simulink model "DLCReferenceApplication"  (R2020b)
settings: Solver=ode23tb  StartTime=0.0  StopTime=25  FixedStep=.001  RelTol=5e-3  EnableMultiTasking=on
StartFcn:
  | %tic
StopFcn:
  | %toc
model workspace (MAT data in the model file):
  DLCXref = [0 7.23 7.5 18 33 33.5 45 50 60]
  DLCYref = [0 0 -4.5 -4 -3.75 1.5 1.25 0 0]
  Downshift_Speeds = [9.5625 12.9375 16.3125 19.6875 23.0625 26.4375 29.8125 33.1875 36.5625 39.9375 43.3125 46.6875 ... (28 elements, 4x7)]
  EngRevLim = 7000
  Pedal_Positions = [0.1 0.4 0.5 0.9]
  Upshift_Speeds = [12.9375 16.3125 19.6875 33 26.4375 29.8125 33.1875 52.5 39.9375 43.3125 46.6875 77.25 ... (28 elements, 4x7)]
  VEH : object (value not decoded)
values from neighbouring files (symbols this model uses):
  L = 3.705    [AOTDataDictionary.sldd]
symbols that are objects in the model workspace (value not decoded): VEH
libraries: simulink x11, autolibutils x4, sim3dlib x2, pid_lib x1, autolibshared x1, vehdynlibdriver x1, vehdynlibscenariocommon x1, vehdynlibsens x1, sim3dautolib x1, vehdynlibviscommon x1
(part 3 of 3)

== system DLCReferenceApplication/Controllers/Transmission Controller/Transmission Controller/TCM/TCM Shift Controller/calc ==
  note: Determine if next gear will be
      | higher or lower than current gear
  gear : Inport
  pedal : Inport  Port=2
  speed : Inport  Port=3
  f : TriggerPort  TriggerType=function-call  VariantControl=Variant  StatesWhenEnabling=reset
      settings: CopyFcn=Stateflow.SLINSF.SimulinkMan.removeBlockPreDeleteFcn  PreDeleteFcn=Stateflow.SLINSF.SimulinkMan.unsafePredeleteFcn
  Add1 : Sum  Inputs=+-
  Add3 : Sum  Inputs=+-
  Add4 : Sum  Inputs=+-
  Calculate Upshift Threshold : Lookup_n-D  BreakpointsForDimension1=Pedal_Positions  BreakpointsForDimension2=1:7  Table=Upshift_Speeds  ExtrapMethod=Clip  UseLastTableValue=on  InternalRulePriority=Speed  RndMeth=Simplest  InputSameDT=on
      settings: InputPortMap=u0,u1
  Calculate Downshift Threshold : Lookup_n-D  BreakpointsForDimension1=Pedal_Positions  BreakpointsForDimension2=2:8  Table=Downshift_Speeds  ExtrapMethod=Clip  UseLastTableValue=on  InternalRulePriority=Speed  RndMeth=Simplest  InputSameDT=on
      settings: InputPortMap=u0,u1
  SpdThr : Outport  VectorParamsAs1DForOutWhenUnconnected=off
  wires:
  pedal/1 -> Calculate Downshift Threshold/1, Calculate Upshift Threshold/1
  gear/1 -> Calculate Downshift Threshold/2, Calculate Upshift Threshold/2
  Calculate Downshift Threshold/1 -> Add3/2
  Calculate Upshift Threshold/1 -> Add1/1
  speed/1 -> Add1/2, Add3/1
  Add1/1 -> Add4/1
  Add3/1 -> Add4/2
  Add4/1 -> SpdThr/1

== system DLCReferenceApplication/Controllers/Transmission Controller/Transmission Controller/TCM/TCM Shift Controller/calc_down ==
  gear : Inport
  pedal : Inport  Port=2
  f : TriggerPort  TriggerType=function-call  VariantControl=Variant  StatesWhenEnabling=reset
      settings: CopyFcn=Stateflow.SLINSF.SimulinkMan.removeBlockPreDeleteFcn  PreDeleteFcn=Stateflow.SLINSF.SimulinkMan.unsafePredeleteFcn
  Calculate Downshift Threshold : Lookup_n-D  BreakpointsForDimension1=Pedal_Positions  BreakpointsForDimension2=2:8  Table=Downshift_Speeds  ExtrapMethod=Clip  UseLastTableValue=on  InternalRulePriority=Speed  RndMeth=Simplest  InputSameDT=on
      settings: InputPortMap=u0,u1
  down_th : Outport  VectorParamsAs1DForOutWhenUnconnected=off
  wires:
  Calculate Downshift Threshold/1 -> down_th/1
  gear/1 -> Calculate Downshift Threshold/2
  pedal/1 -> Calculate Downshift Threshold/1

== system DLCReferenceApplication/Controllers/Transmission Controller/Transmission Controller/TCM/TCM Shift Controller/calc_up ==
  gear : Inport
  pedal : Inport  Port=2
  f : TriggerPort  TriggerType=function-call  VariantControl=Variant  StatesWhenEnabling=reset
      settings: CopyFcn=Stateflow.SLINSF.SimulinkMan.removeBlockPreDeleteFcn  PreDeleteFcn=Stateflow.SLINSF.SimulinkMan.unsafePredeleteFcn
  Calculate Upshift Threshold : Lookup_n-D  BreakpointsForDimension1=Pedal_Positions  BreakpointsForDimension2=1:7  Table=Upshift_Speeds  ExtrapMethod=Clip  UseLastTableValue=on  InternalRulePriority=Speed  RndMeth=Simplest  InputSameDT=on
      settings: InputPortMap=u0,u1
  up_th : Outport  VectorParamsAs1DForOutWhenUnconnected=off
  wires:
  Calculate Upshift Threshold/1 -> up_th/1
  pedal/1 -> Calculate Upshift Threshold/1
  gear/1 -> Calculate Upshift Threshold/2

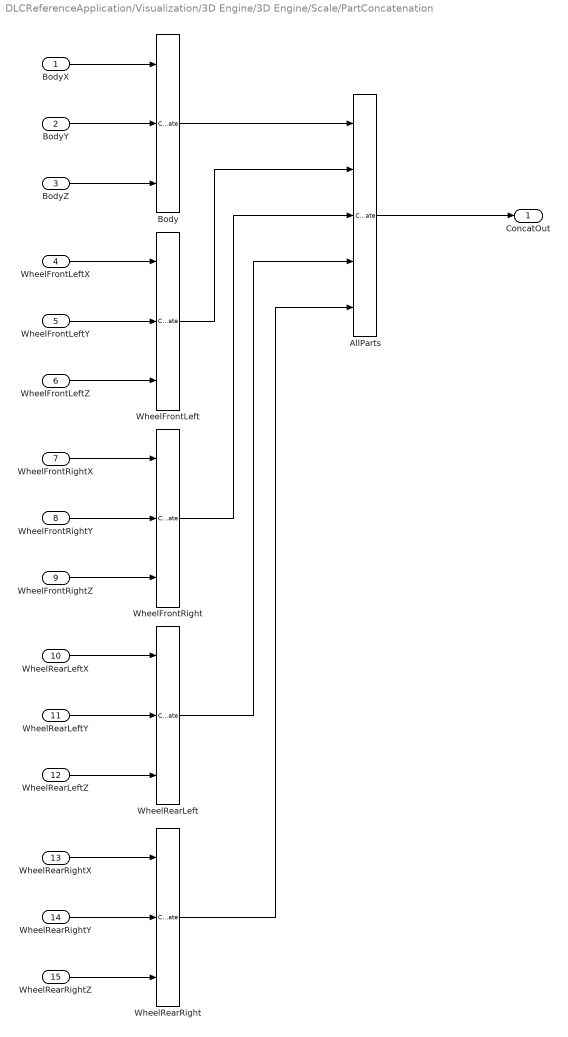
== system DLCReferenceApplication/Visualization/3D Engine/3D Engine/Scale/PartConcatenation ==
  BodyX : Inport
  BodyY : Inport  Port=2
  BodyZ : Inport  Port=3
  WheelFrontLeftX : Inport  Port=4
  WheelFrontLeftY : Inport  Port=5
  WheelFrontLeftZ : Inport  Port=6
  WheelFrontRightX : Inport  Port=7
  WheelFrontRightY : Inport  Port=8
  WheelFrontRightZ : Inport  Port=9
  WheelRearLeftX : Inport  Port=10
  WheelRearLeftY : Inport  Port=11
  WheelRearLeftZ : Inport  Port=12
  WheelRearRightX : Inport  Port=13
  WheelRearRightY : Inport  Port=14
  WheelRearRightZ : Inport  Port=15
  AllParts : Concatenate  NumInputs=5  Mode=Multidimensional array
  Body : Concatenate  NumInputs=3  Mode=Multidimensional array  ConcatenateDimension=2
  WheelFrontLeft : Concatenate  NumInputs=3  Mode=Multidimensional array  ConcatenateDimension=2
  WheelFrontRight : Concatenate  NumInputs=3  Mode=Multidimensional array  ConcatenateDimension=2
  WheelRearLeft : Concatenate  NumInputs=3  Mode=Multidimensional array  ConcatenateDimension=2
  WheelRearRight : Concatenate  NumInputs=3  Mode=Multidimensional array  ConcatenateDimension=2
  ConcatOut : Outport  VectorParamsAs1DForOutWhenUnconnected=off
  wires:
  BodyX/1 -> Body/1
  BodyZ/1 -> Body/3
  WheelFrontLeftX/1 -> WheelFrontLeft/1
  WheelFrontLeftZ/1 -> WheelFrontLeft/3
  WheelFrontLeftY/1 -> WheelFrontLeft/2
  BodyY/1 -> Body/2
  WheelFrontLeft/1 -> AllParts/2
  WheelRearRightX/1 -> WheelRearRight/1
  Body/1 -> AllParts/1
  WheelRearLeft/1 -> AllParts/4
  WheelFrontRight/1 -> AllParts/3
  WheelRearRightZ/1 -> WheelRearRight/3
  WheelFrontRightY/1 -> WheelFrontRight/2
  WheelFrontRightX/1 -> WheelFrontRight/1
  WheelRearRightY/1 -> WheelRearRight/2
  WheelRearLeftZ/1 -> WheelRearLeft/3
  AllParts/1 -> ConcatOut/1
  WheelRearLeftY/1 -> WheelRearLeft/2
  WheelRearRight/1 -> AllParts/5
  WheelRearLeftX/1 -> WheelRearLeft/1
  WheelFrontRightZ/1 -> WheelFrontRight/3

== stateflow chart DLCReferenceApplication/Controllers/Transmission Controller/Transmission Controller/TCM/TCM Shift Controller ==
  settings: sampleTime=0.01
  state GearCmd [parallel]
    settings: executionOrder=1
    state Neutral
      en:
      GearCmd = 0;
    state G1
      en:
      GearCmd = 1;
    state G2
      en:
      GearCmd = 2;
      du:
      [SpdThr] = calc(2,pedal,speed);
    state G3
      en:
      GearCmd = 3;
      du:
      [SpdThr] = calc(3,pedal,speed);
    state G8
      en:
      GearCmd = 8;
    state G7
      en:
      GearCmd = 7;
    state G6
      en:
      GearCmd = 6;
    state G5
      en:GearCmd=5;
      du:[SpdThr]=calc(5,pedal,speed);
    state G4
      en:
      GearCmd = 4;
      du:
      [SpdThr] = calc(4,pedal,speed);
    (default) -> Neutral
    Neutral -> G1 : [~Neutral]
    G1 -> G2 [order 1] : Up
    G2 -> G3 [order 1] : Up
    G1 -> Neutral [order 2] : [Neutral]
    G2 -> G1 [order 2] : Down
    G3 -> G2 [order 2] : Down
    G3 -> G4 [order 1] : Up
    G4 -> G3 [order 2] : Down
    G7 -> G8 [order 1] : Up
    G5 -> G6 [order 1] : Up
    G6 -> G7 [order 1] : Up
    G4 -> G5 [order 1] : Up
    G5 -> G4 [order 2] : Down
    G6 -> G5 [order 2] : Down
    G7 -> G6 [order 2] : Down
    G8 -> G7 : Down
  state SelectionState [parallel]
    du:[up_th]=calc_up(GearCmd,pedal);
    du:[down_th]=calc_down(GearCmd,pedal);
    settings: executionOrder=2
    state SteadyState
      en:
      clutchControl = 0;
    state preDownShifting
    state preUpShifting
    state UpShifting
      en:
      GearCmd = GearCmd + 0.5;
    state DownShifting
      en:
      GearCmd = GearCmd - 0.5;
    (default) -> SteadyState
    SteadyState -> (junction 62) [order 1] : [speed < down_th && ...
        | GearCmd >1]
    SteadyState -> (junction 128) [order 2] : [speed > up_th &&...
        | GearCmd <= 5 && ...
        | floor(GearCmd) == GearCmd]
    (junction 62) -> preDownShifting
    (junction 128) -> preUpShifting
    (junction 168) -> SteadyState
    (junction 23) -> SteadyState
    (junction 161) -> SteadyState
    preDownShifting -> (junction 168) [order 2] : [speed >= down_th]
    preUpShifting -> (junction 161) [order 2] : [speed <= up_th]
    preUpShifting -> UpShifting [order 1] : after(0.5,sec)
        | [speed>up_th]
    preDownShifting -> DownShifting [order 1] : after(0.5, sec)
        | [speed < down_th - 2]
    DownShifting -> (junction 23) : {GearCmd.Down;}
    UpShifting -> (junction 23) : {GearCmd.Up;}
  state up_th = calc_up(gear,pedal) [function]
  state down_th = calc_down(gear,pedal) [function]
  state SpdThr = calc(gear,pedal,speed) [function]
  data: gear function_input; pedal function_input; up_th function_output; gear function_input; pedal function_input; down_th function_output; gear function_input; pedal function_input; SpdThr function_output; speed function_input; GearCmd output int8; speed input; pedal input; clutchControl local double; SpdThr local double; Neutral input; up_th local double; down_th local double
  events: Up local EITHER_EDGE_EVENT; Down local EITHER_EDGE_EVENT

== stateflow chart DLCReferenceApplication/Controllers/Transmission Controller/PRNDL Controller/Shift Controller ==
  settings: sampleTime=0.01
  state GearSelect [parallel]
    settings: executionOrder=1
    state Reverse
      entry:
      GearState = -1;
    state Neutral
      entry:
      GearState = 0;
    state Odd
      en:GearState = Gear;
      du:[SpdThr]=calc(Gear,Accel,VehVel);
    state Even
      en:GearState = Gear;
      du:[SpdThr]=calc(Gear,Accel,VehVel);
    state Park
      entry:
      GearState = 80;
    (default) -> (junction 461) : /* InitialGear */
        | {Gear = GearInit;}
    (junction 461) -> (junction 463) [order 1] : [GearInit==80]
    (junction 463) -> Park
    (junction 461) -> (junction 441) [order 2]
    (junction 441) -> (junction 442) [order 1] : [GearInit<0]
    (junction 442) -> Reverse
    (junction 441) -> (junction 457) [order 2]
    (junction 457) -> (junction 459) [order 1] : [GearInit==0]
    (junction 459) -> Neutral
    (junction 457) -> (junction 445) [order 2]
    (junction 445) -> (junction 446) [order 1] : [GearInit%%2==0]
    (junction 445) -> Odd [order 2]
    (junction 446) -> Even
    (junction 363) -> (junction 366)
    (junction 366) -> Odd
    Even -> (junction 363) [order 1] : UP
        | {Gear=Gear+1;}
    Neutral -> Reverse [order 2] : [PRNDL==-1]
        | {Gear=-1;}
    Neutral -> Odd [order 1] : UP
        | {Gear=Gear+1;}
    Odd -> Even [order 1] : UP
        | {Gear=Gear+1;}
    Reverse -> Neutral : [PRNDL==1]
        | {Gear=1;}
    Even -> Odd [order 2] : DOWN
        | {Gear=Gear-1;}
    Neutral -> (junction 380) [order 3]
    (junction 379) -> Neutral
    (junction 370) -> Neutral
    Odd -> (junction 361) [order 2] : DOWN
        | {Gear=Gear-1;}
    (junction 357) -> Even
    Even -> (junction 371) [order 3] : [Gear==0]
    (junction 361) -> (junction 357)
    (junction 380) -> Park : after(tPark,sec)
        | [PRNDL==80 &&...
        | Brake>0.5&&...
        | abs(VehVel)<=1&&...
        | Accel<=0.05]
    Park -> (junction 379) : [abs(VehVel)<=1&&Accel>0]
    (junction 371) -> (junction 370)
  state SelectionState [parallel]
    du:[up_th]=calc_up(GearState,Accel);
    du:[down_th]=calc_down(GearState,Accel);
    settings: executionOrder=2
    state Inactive
    state SteadyState
      en:
      clutchControl = 0;
    state preUpShifting
      en:clutchControl = 1;
    state preDownShifting
      en:clutchControl = 1;
    state UpShifting
      en:
      GearState = GearState + 0.5;
    state DownShifting
      en:
      GearState = GearState - 0.5;
    (default) -> (junction 514)
    (junction 514) -> Inactive [order 2]
    (junction 514) -> SteadyState [order 1] : [PRNDL==1]
    (junction 517) -> Inactive
    Inactive -> (junction 520) : [PRNDL==1]
    SteadyState -> (junction 517) [order 3] : [PRNDL~=1]
    SteadyState -> (junction 62) [order 2] : [GearState >0&&...
        | (VehVel < down_th ||...
        |  EngSpd<1200)]
    (junction 62) -> preDownShifting
    (junction 520) -> SteadyState
    SteadyState -> (junction 128) [order 1] : [Accel>0 && (abs(VehVel) > up_th) &&...
        | (GearState <= N ) &&...
        | (floor(GearState) == GearState) &&...
        | (EngSpd>=2000)]
    (junction 128) -> preUpShifting
    (junction 168) -> SteadyState
    (junction 23) -> SteadyState
    (junction 161) -> SteadyState
    preDownShifting -> (junction 168) [order 2] : [VehVel >= down_th &&...
        | EngSpd>2000]
    preUpShifting -> (junction 161) [order 2] : [VehVel <= up_th ||...
        |  EngSpd<1200]
    preUpShifting -> UpShifting [order 1] : after(tClutch,sec)
        | [VehVel>up_th]
    preDownShifting -> DownShifting [order 1] : after(tClutch, sec)
        | [(VehVel < down_th - 2) || VehVel<=0 ||EngSpd<750]
    DownShifting -> (junction 23) : {GearSelect.DOWN;}
    UpShifting -> (junction 23) : {GearSelect.UP;}
  state up_th = calc_up(Gear,Accel) [function]
  state down_th = calc_down(Gear,Accel) [function]
  state SpdThr = calc(Gear,pedal,VehVel) [function]
  data: Gear function_input; Accel function_input; up_th function_output; Gear function_input; Accel function_input; down_th function_output; Gear function_input; pedal function_input; SpdThr function_output; VehVel function_input; PRNDL input; Gear output double =GearInit; clutchControl output double; Accel input; Brake input; EngSpd input; VehVel input; SpdThr local double; up_th local double; down_th local double; tPark parameter; tRev parameter; GearInit parameter double; N local double =size(upShftTbl,2); tClutch parameter; GearState local double
  events: DOWN local EITHER_EDGE_EVENT; UP local EITHER_EDGE_EVENT
